simulink model "ParkSensor"  (R2016b)
settings: Solver=VariableStepAuto  StartTime=0.0  StopTime=inf  RelTol=1e-3
libraries: simulink x1
settings Model: Creator=Stefano  LastModifiedBy=Michele
settings OptimizationCC: DefaultParameterBehavior=Inlined
settings DebuggingCC: ParameterTunabilityLossMsg=error
settings RTWCC: SystemTargetFile=ert.tlc  TemplateMakefile=ert_default_tmf  Description=Embedded Coder  GenerateReport=on  IncludeHyperlinkInReport=on  LaunchReport=on  GenerateTraceInfo=on  GenerateTraceReport=on  GenerateTraceReportSl=on  GenerateTraceReportSf=on  GenerateTraceReportEml=on  GenerateCodeMetricsReport=on
settings CodeAppCC: ForceParamTrailComments=on  IgnoreCustomStorageClasses=off  OperatorAnnotations=on  SimulinkDataObjDesc=on  SFDataObjDesc=on  MATLABFcnDesc=on  InsertBlockDesc=on  MATLABSourceComments=on
settings ERTTargetCC: TargetLangStandard=C99 (ISO)  GenerateSampleERTMain=on  SupportAbsoluteTime=off  MultiInstanceERTCode=on  CodeInterfacePackaging=Reusable function  SupportNonFinite=off  SupportComplex=off  InlinedParameterPlacement=NonHierarchical  MultiInstanceErrorCode=None  ERTCustomFileTemplate=example_file_process.tlc

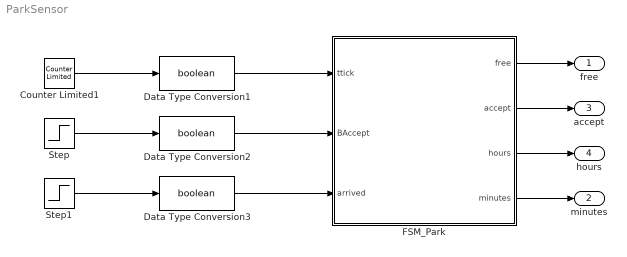
== system ParkSensor ==
  Counter Limited1 : simulink/Sources/Counter Limited  uplimit=1  tsamp=0.1
  Data Type Conversion1 : DataTypeConversion  OutDataTypeStr=boolean
  Data Type Conversion2 : DataTypeConversion  OutDataTypeStr=boolean
  Data Type Conversion3 : DataTypeConversion  OutDataTypeStr=boolean
  FSM_Park : Subsystem
  Step : Step  SampleTime=0.1
  Step1 : Step  Time=2  SampleTime=0.1
  free : Outport
  minutes : Outport  Port=2
  accept : Outport  Port=3
  hours : Outport  Port=4
  wires:
  Counter Limited1/1 -> Data Type Conversion1/1
  Data Type Conversion1/1 -> FSM_Park/1(ttick)
  FSM_Park/1(free) -> free/1
  FSM_Park/4(minutes) -> minutes/1
  FSM_Park/3(hours) -> hours/1
  FSM_Park/2(accept) -> accept/1
  Step1/1 -> Data Type Conversion3/1
  Step/1 -> Data Type Conversion2/1
  Data Type Conversion2/1 -> FSM_Park/2(BAccept)
  Data Type Conversion3/1 -> FSM_Park/3(arrived)

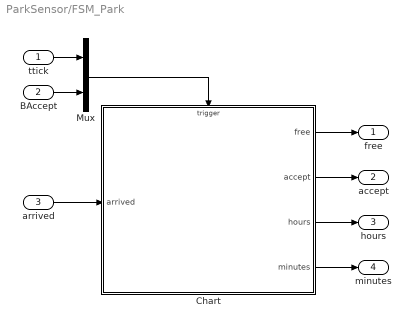
== system ParkSensor/FSM_Park ==
  ttick : Inport
  BAccept : Inport  Port=2
  arrived : Inport  Port=3
  Chart : Stateflow chart  TreatAsAtomicUnit=on
  Mux : Mux  Inputs=2
  free : Outport
  accept : Outport  Port=2
  hours : Outport  Port=3
  minutes : Outport  Port=4
  wires:
  arrived/1 -> Chart/1(arrived)
  Chart/1(free) -> free/1
  Chart/2(accept) -> accept/1
  Chart/3(hours) -> hours/1
  Chart/4(minutes) -> minutes/1
  Mux/1 -> Chart/Trigger
  ttick/1 -> Mux/1
  BAccept/1 -> Mux/2

== stateflow chart ParkSensor/FSM_Park/Chart ==
  settings: executeAtInitialization=1
  state control [parallel]
    settings: executionOrder=1
    state Free
    state Accept_Arrivals
      en: accept = true
      ex: accept = false
    state Parked
      en: free = false
    state Accept_Departure
      en: accept = true;
      ex: accept = false;
      free = true;
    (default) -> Free : {free = true; accept = false}
    Free -> Accept_Arrivals : [arrived==true]
    Accept_Arrivals -> Free [order 2] : [arrived == false]
    Accept_Departure -> Accept_Arrivals [order 2] : BAccept[arrived == true]
    Accept_Arrivals -> Parked [order 1] : BAccept/{hours = uint8(0);
        | minutes = uint8(0)}
    Accept_Departure -> Free [order 1] : BAccept/{hours = uint8(0);
        | minutes = uint8(0)}
    Parked -> Accept_Departure : [arrived==false]
  state time [parallel]
    settings: executionOrder=2
    state timecount
    (default) -> timecount : /{hours=uint8(0);minutes=uint8(0);seconds=uint8(0);}
    timecount -> (junction 104) : ttick {seconds=mod(seconds+1,60)}
    (junction 104) -> (junction 109) [order 2]
    (junction 104) -> (junction 103) [order 1] : [seconds==0]{minutes=mod(minutes+1, 60)}
    (junction 109) -> timecount
    (junction 103) -> (junction 109) [order 2]
    (junction 103) -> timecount [order 1] : [minutes==0]{hours=mod(hours+1,24)}
  data: free output boolean; accept output boolean; hours output uint8; minutes output uint8; arrived input boolean; seconds local uint8
  events: ttick input RISING_EDGE_EVENT; BAccept input RISING_EDGE_EVENT
